simulink model "ex3_model"  (R2024b)
settings: Solver=ode45  StartTime=0.0  StopTime=5  MaxStep=1.0E-3  RelTol=1e-5
values from neighbouring files (symbols this model uses):
  A = [0 1; -2 -40]    [ex3.m]
  Ao = sysd.A - L*sysd.C    [ex3.m]
  Aod = sysd.A(2,2) - Ld*sysd.A(1,2)    [ex3.m]
  B = [0; 40]    [ex3.m]
  Bo = [sysd.B, L]    [ex3.m]
  Bod = [sysd.B(2) - Ld*sysd.B(1), Aod*Ld + sysd.A(2,1) - Ld*sysd.A(1,1)]    [ex3.m]
  C = [1 0]    [ex3.m]
  Co = eye(2,2)    [ex3.m]
  Cod = [0;1]    [ex3.m]
  D = 0    [ex3.m]
  Do = zeros(2,2)    [ex3.m]
  Dod = [0 1; 0 Ld]    [ex3.m]
  K = K(2:end)    [ex3.m]
  Ki = K(1)    [ex3.m]
  Nu = ff_gains(3)    [ex3.m]
  Nx = ff_gains(1:2)    [ex3.m]
  Ts = 0.01*1e-3    (= 1e-05)    [ex3.m]
undefined symbols (not defined in the file or in its folder): DiscIntNeverNeededParam
settings Model: Creator=Nihal  LastModifiedBy=pries

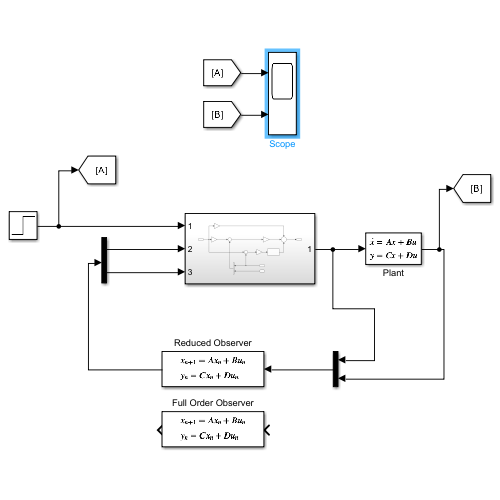
[thumbnail: Simulink's stored preview of the top-level diagram]
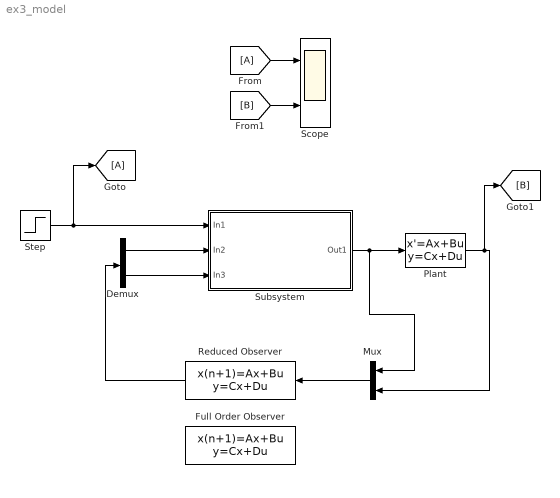
== system ex3_model ==
  Demux : Demux  Outputs=2
  From : From
  Full Order Observer : DiscreteStateSpace  A=Ao  B=Bo  C=Co  D=Do  SampleTime=Ts
  Goto : Goto
  Mux : Mux  Inputs=2
  Plant : StateSpace  A=A  B=B  C=C  D=D  InitialCondition=0
  Reduced Observer : DiscreteStateSpace  A=Aod  B=Bod  C=Cod  D=Dod  SampleTime=Ts
  Scope : Scope  NumInputPorts=2
  Step : Step  After=40  SampleTime=0
  Subsystem : Subsystem
  wires:
  Demux/1 -> Subsystem/2(In2)
  Demux/2 -> Subsystem/3(In3)
  Step/1 -> Goto/1, Subsystem/1(In1)
  Subsystem/1(Out1) -> Mux/1, Plant/1
  Plant/1 -> [B], Mux/2
  From/1 -> Scope/1
  [B] -> Scope/2
  Mux/1 -> Reduced Observer/1
  Reduced Observer/1 -> Demux/1

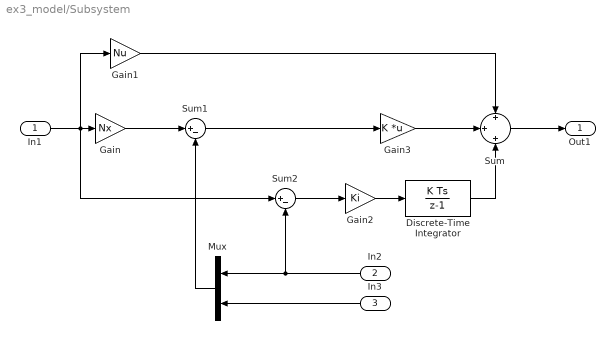
== system ex3_model/Subsystem ==
  In1 : Inport
  In2 : Inport  Port=2
  In3 : Inport  Port=3
  Discrete-Time Integrator : DiscreteIntegrator  SampleTime=Ts  ICPrevOutput=DiscIntNeverNeededParam  ICPrevScaledInput=DiscIntNeverNeededParam
  Gain : Gain  Gain=Nx
  Gain1 : Gain  Gain=Nu
  Gain2 : Gain  Gain=Ki
  Gain3 : Gain  Gain=K  Multiplication=Matrix(K*u)
  Mux : Mux  Inputs=2
  Sum : Sum  Inputs=+|+|+
  Sum1 : Sum  Inputs=|+-
  Sum2 : Sum  Inputs=|+-
  Out1 : Outport
  wires:
  In3/1 -> Mux/2
  In2/1 -> Sum2/2, Mux/1
  Gain/1 -> Sum1/1
  Gain1/1 -> Sum/1
  Sum1/1 -> Gain3/1
  In1/1 -> Sum2/1, Gain1/1, Gain/1
  Gain3/1 -> Sum/2
  Mux/1 -> Sum1/2
  Sum/1 -> Out1/1
  Sum2/1 -> Gain2/1
  Gain2/1 -> Discrete-Time Integrator/1
  Discrete-Time Integrator/1 -> Sum/3
